simulink model "text009"  (R2020b)
settings: Solver=VariableStepAuto  StartTime=0.0  StopTime=10.0  RelTol=1e-3
libraries: powerlib x15, eeDiscretePi x2, powerlib_extras x2
settings Model: Creator=38061  LastModifiedBy=38061

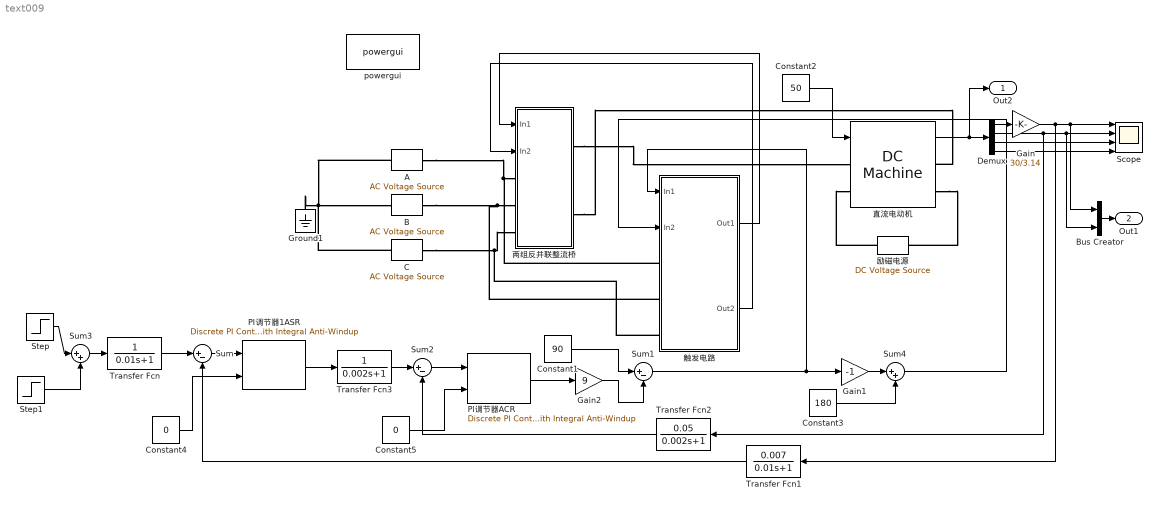
== system text009 ==
  A : powerlib/Electrical Sources/AC Voltage Source  Amplitude=220  Phase=0  Frequency=50  SampleTime=0  Measurements=None  BusType=swing  Pref=10e3  Qref=0  Qmin=-inf  Qmax=+inf
  B : powerlib/Electrical Sources/AC Voltage Source  Amplitude=220  Phase=120  Frequency=50  SampleTime=0  Measurements=None  BusType=swing  Pref=10e3  Qref=0  Qmin=-inf  Qmax=+inf
  Bus Creator : BusCreator  Inputs=2
  C : powerlib/Electrical Sources/AC Voltage Source  Amplitude=220  Phase=240  Frequency=50  SampleTime=0  Measurements=None  BusType=swing  Pref=10e3  Qref=0  Qmin=-inf  Qmax=+inf
  Constant1 : Constant  Value=90
  Constant2 : Constant  Value=50
  Constant3 : Constant  Value=180
  Constant4 : Constant  Value=0
  Constant5 : Constant  Value=0
  Demux : Demux
  Gain : Gain  Gain=30/3.14
  Gain1 : Gain  Gain=-1
  Gain2 : Gain  Gain=9
  Ground1 : powerlib/Elements/Ground  LConnTagsString=a
  PI调节器1ASR : eeDiscretePi/Discrete PI Controller with Integral Anti-Windup  Kp=11.7  Ki=134.4  x0=0  B=10  A=0  Ts=50e-6
      settings: SourceProductBaseCode=PS
  PI调节器ACR : eeDiscretePi/Discrete PI Controller with Integral Anti-Windup  Kp=1.013  Ki=33.76  x0=0  B=10  A=-10  Ts=50e-6
      settings: SourceProductBaseCode=PS
  Scope : Scope  NumInputPorts=4
  Step : Step  Time=0  After=10  SampleTime=0
  Step1 : Step  Time=1.5  After=-20  SampleTime=10
  Sum : Sum  Inputs=|+-
  Sum1 : Sum  Inputs=|+-
  Sum2 : Sum  Inputs=|+-
  Sum3 : Sum  Inputs=|++
  Sum4 : Sum  Inputs=|++
  Transfer Fcn : TransferFcn  Denominator=[0.01 1]
  Transfer Fcn1 : TransferFcn  Numerator=[0.007]  Denominator=[0.01 1]
  Transfer Fcn2 : TransferFcn  Numerator=[0.05]  Denominator=[0.002 1]
  Transfer Fcn3 : TransferFcn  Denominator=[0.002 1]
  powergui : powerlib/powergui  Priority=1  SimulationMode=Continuous  SampleTime=50e-6  frequency=60  Iterations=50  frequencyindice=50  Pbase=100e6  ErrMax=1e-4  UnitsV=kV  UnitsW=MW  buscounter=0  FunctionMessages=off  echomessages=off  EnableUseOfTLC=off  CurrentSourceSwitches=off  DisableSnubberDevices=off  DisableRonSwitches=off  DisableVfSwitches=off  DisplayEquations=off  AutomaticDiscreteSolvers=off  SolverType=Tustin/Backward Euler (TBE)  Interpol=off  ExternalGateDelay=off  methode=off  Ts=100  x0status=blocks  SPID=on  SwTol=0  HookPort=off  NonlinearTolerance=1e-4  nMaxIteration=100  ContinueOnMaxIteration=off  RestoreLinks=warning  ResistiveCurrentMeasurement=off  Frange=[0:2:500]  Ylog=off  Xlog=on  ShowGrid=off  save=off  variable=ZData  structure=0  ZoomFFT=off  StartTime=0.0  cycles=1  DisplayStyle=1  fundamental=60  FreqAxis=off  MaxFrequency=1000  frequencyindicesteady=1  RmsSteady=1  display=off
  两组反并联整流桥 : Subsystem
  励磁电源 : powerlib/Electrical Sources/DC Voltage Source  Amplitude=220  Measurements=None
  直流电动机 : powerlib/Machines/DC Machine  PresetModel=No  MechanicalLoad=Torque TL  FieldType=Wound  ShowDetailedParameters=on  MeasurementBus=off  RLa="[ 0.5  0.017]"  RLf="[ 240  120]"  Laf=2  MachineConstant=Torque constant (N.m/A)  Ke=1.8  Kt=1.8  J=0.255  Bm=0  Tf=0  w0=1  Ifinit=0.916666666666667  TsPowergui=0  TsBlock=-1
  触发电路 : Subsystem
  Out2 : Outport
  Out1 : Outport  Port=2
  wires:
  Bus Creator/1 -> Out1/1
  Transfer Fcn2/1 -> Sum2/2
  Gain/1 -> Transfer Fcn1/1, Bus Creator/1, Scope/1
  Demux/2 -> Transfer Fcn2/1, Bus Creator/2, Scope/2
  PI调节器ACR/1 -> Gain2/1
  Demux/3 -> Scope/3
  Gain2/1 -> Sum1/2
  PI调节器1ASR/1 -> Transfer Fcn3/1
  Demux/1 -> Gain/1
  Constant1/1 -> Sum1/1
  Transfer Fcn1/1 -> Sum/2
  Transfer Fcn3/1 -> Sum2/1
  Sum/1 -> PI调节器1ASR/1
  Sum2/1 -> PI调节器ACR/1
  Transfer Fcn/1 -> Sum/1
  直流电动机/1 -> Out2/1, Demux/1
  Constant2/1 -> 直流电动机/1
  Demux/4 -> Scope/4
  触发电路/1(Out1) -> 两组反并联整流桥/1(In1)
  触发电路/2(Out2) -> 两组反并联整流桥/2(In2)
  Sum3/1 -> Transfer Fcn/1
  Sum1/1 -> Gain1/1, 触发电路/1(In1)
  Gain1/1 -> Sum4/1
  Constant3/1 -> Sum4/2
  Sum4/1 -> 触发电路/2(In2)
  Step/1 -> Sum3/1
  Step1/1 -> Sum3/2
  Constant5/1 -> PI调节器ACR/2
  Constant4/1 -> PI调节器1ASR/2
  connections:
  B/RConn1 -- 触发电路/LConn2 -- 两组反并联整流桥/LConn2
  C/RConn1 -- 触发电路/LConn3 -- 两组反并联整流桥/LConn3
  A/RConn1 -- 触发电路/LConn1 -- 两组反并联整流桥/LConn1
  Ground1/LConn1 -- C/LConn1 -- A/LConn1 -- B/LConn1
  励磁电源/RConn1 -- 直流电动机/LConn2
  直流电动机/RConn2 -- 励磁电源/LConn1
  两组反并联整流桥/RConn1 -- 直流电动机/LConn1
  两组反并联整流桥/RConn2 -- 直流电动机/RConn1

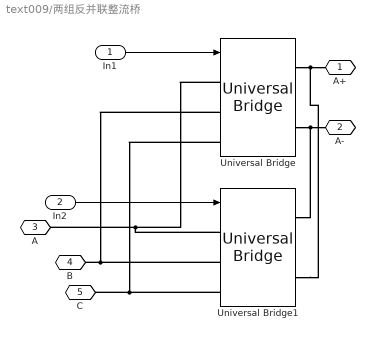
== system text009/两组反并联整流桥 ==
  In1 : Inport
  In2 : Inport  Port=2
  Universal Bridge : powerlib/Power Electronics/Universal Bridge  Arms=3  SnubberResistance=1e5  SnubberCapacitance=inf  Device=Thyristors  Ron=1e-3  Lon=0  ForwardVoltages="[  0  0  ]"  ForwardVoltage=0  GTOparameters=[ 10e-6 , 20e-6 ]  IGBTparameters=[ 1e-6 , 2e-6 ]  Measurements=None  Measurements_2=None  converterType=Rectifier
  Universal Bridge1 : powerlib/Power Electronics/Universal Bridge  Arms=3  SnubberResistance=1e5  SnubberCapacitance=inf  Device=Thyristors  Ron=1e-3  Lon=0  ForwardVoltages="[  0  0  ]"  ForwardVoltage=0  GTOparameters=[ 10e-6 , 20e-6 ]  IGBTparameters=[ 1e-6 , 2e-6 ]  Measurements=None  Measurements_2=None  converterType=Rectifier
  A+ : PMIOPort  Side=Right
  A- : PMIOPort  Port=2  Side=Right
  A : PMIOPort  Port=3  Side=Left
  B : PMIOPort  Port=4  Side=Left
  C : PMIOPort  Port=5  Side=Left
  wires:
  In1/1 -> Universal Bridge/1
  In2/1 -> Universal Bridge1/1
  connections:
  Universal Bridge1/LConn1 -- A/RConn1 -- Universal Bridge/LConn1
  Universal Bridge1/LConn2 -- Universal Bridge/LConn2 -- B/RConn1
  Universal Bridge/RConn1 -- Universal Bridge1/RConn2 -- A+/RConn1
  Universal Bridge/RConn2 -- Universal Bridge1/RConn1 -- A-/RConn1
  Universal Bridge1/LConn3 -- Universal Bridge/LConn3 -- C/RConn1

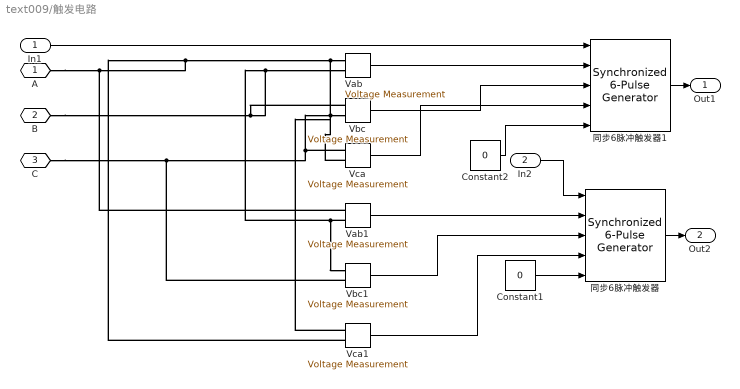
== system text009/触发电路 ==
  In1 : Inport
  In2 : Inport  Port=2
  Constant1 : Constant  Value=0
  Constant2 : Constant  Value=0
  Vab : powerlib/Measurements/Voltage Measurement  PhasorSimulation=off  OutputType=Complex  PSBequivalent=0
  Vab1 : powerlib/Measurements/Voltage Measurement  PhasorSimulation=off  OutputType=Complex  PSBequivalent=0
  Vbc : powerlib/Measurements/Voltage Measurement  PhasorSimulation=off  OutputType=Complex  PSBequivalent=0
  Vbc1 : powerlib/Measurements/Voltage Measurement  PhasorSimulation=off  OutputType=Complex  PSBequivalent=0
  Vca : powerlib/Measurements/Voltage Measurement  PhasorSimulation=off  OutputType=Complex  PSBequivalent=0
  Vca1 : powerlib/Measurements/Voltage Measurement  PhasorSimulation=off  OutputType=Complex  PSBequivalent=0
  同步6脉冲触发器 : powerlib_extras/Control  Blocks/Synchronized 6-Pulse Generator  freq=50  pwidth=10  Double_Pulse=off
      settings: SourceProductBaseCode=PS
  同步6脉冲触发器1 : powerlib_extras/Control  Blocks/Synchronized 6-Pulse Generator  freq=50  pwidth=10  Double_Pulse=off
      settings: SourceProductBaseCode=PS
  A : PMIOPort  Side=Left
  B : PMIOPort  Port=2  Side=Left
  C : PMIOPort  Port=3  Side=Left
  Out1 : Outport
  Out2 : Outport  Port=2
  wires:
  In2/1 -> 同步6脉冲触发器/1
  In1/1 -> 同步6脉冲触发器1/1
  同步6脉冲触发器1/1 -> Out1/1
  同步6脉冲触发器/1 -> Out2/1
  Constant2/1 -> 同步6脉冲触发器1/5
  Constant1/1 -> 同步6脉冲触发器/5
  Vab/1 -> 同步6脉冲触发器1/2
  Vbc/1 -> 同步6脉冲触发器1/3
  Vca/1 -> 同步6脉冲触发器1/4
  Vab1/1 -> 同步6脉冲触发器/2
  Vbc1/1 -> 同步6脉冲触发器/3
  Vca1/1 -> 同步6脉冲触发器/4
  connections:
  B/RConn1 -- Vbc/LConn1 -- Vbc1/LConn1 -- Vab1/LConn2 -- Vab/LConn2
  A/RConn1 -- Vab1/LConn1 -- Vab/LConn1 -- Vca/LConn2 -- Vca1/LConn2
  C/RConn1 -- Vbc1/LConn2 -- Vca/LConn1 -- Vca1/LConn1 -- Vbc/LConn2
